simulink model "DCMG_BDCUIO_jan2025_scenario_3"  (R2018b)
settings: Solver=ode1  StartTime=0.0  StopTime=2  FixedStep=1e-6  RelTol=1e-3
undefined symbols (not defined in the file): Cdc, Cpv, dEgdT, EgRef, gcbh, k1, KIvp, KPvp, Rsh_array5pc, sigbuilder_block, sps_rtmsupport, Tref_K, Ts, VT_ref
libraries: powerlib x42, spsPVarrayModel x3
(part 6 of 6)

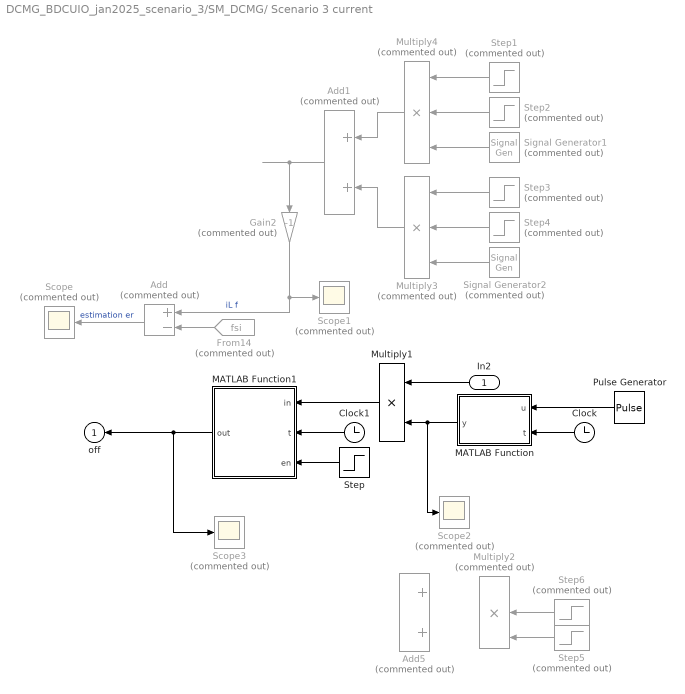
== system DCMG_BDCUIO_jan2025_scenario_3/SM_DCMG/ Scenario 3 current ==
  In2 : Inport
  Add : Sum  Commented=on  Inputs=+-
  Add1 : Sum  Commented=on
  Add5 : Sum  Commented=on
  Clock : Clock
  Clock1 : Clock
  From14 : From  Commented=on  GotoTag=fsi  TagVisibility=global
  Gain2 : Gain  Commented=on  Gain=-1
  MATLAB Function : MATLAB Function  TreatAsAtomicUnit=on
  MATLAB Function1 : MATLAB Function  TreatAsAtomicUnit=on
  Multiply1 : Product
  Multiply2 : Product  Commented=on  Inputs=3
  Multiply3 : Product  Commented=on  Inputs=3
  Multiply4 : Product  Commented=on  Inputs=3
  Pulse Generator : DiscretePulseGenerator  PulseType=Time based  Period=0.01  PulseWidth=40
  Scope{,1..3} (4 alike) : Scope  Commented=on
  Signal Generator1 : SignalGenerator  Commented=on  WaveForm=random  Amplitude=3  Frequency=1100
  Signal Generator2 : SignalGenerator  Commented=on  Amplitude=2  Frequency=25*3.14  Units=rad/sec
  Step : Step  Time=1.1  Before=1  After=0  SampleTime=0
  Step1 : Step  Commented=on  Time=1.1  Before=1  After=0  SampleTime=0
  Step2 : Step  Commented=on  Time=0.7  SampleTime=0
  Step3 : Step  Commented=on  Time=1.7  Before=1  After=0  SampleTime=0
  Step4 : Step  Commented=on  Time=1.2  SampleTime=0
  Step5 : Step  Commented=on  Time=0.5  Before=1  After=0  SampleTime=0
  Step6 : Step  Commented=on  Time=0.25  SampleTime=0
  off : Outport
  wires:
  MATLAB Function/1(y) -> Multiply1/2, Scope2/1
  Clock1/1 -> MATLAB Function1/2(t)
  Step/1 -> MATLAB Function1/3(en)
  MATLAB Function1/1(out) -> off/1, Scope3/1
  Clock/1 -> MATLAB Function/2(t)
  Step6/1 -> Multiply2/2
  Step5/1 -> Multiply2/3
  Pulse Generator/1 -> MATLAB Function/1(u)
  From14/1 -> Add/2
  Add/1 -> Scope/1  "estimation er"
  Signal Generator2/1 -> Multiply3/3
  Step4/1 -> Multiply3/2
  Step3/1 -> Multiply3/1
  Step2/1 -> Multiply4/2
  Step1/1 -> Multiply4/1
  Gain2/1 -> Add/1, Scope1/1  "iL f"
  Add1/1 -> Gain2/1
  Multiply3/1 -> Add1/2
  Multiply4/1 -> Add1/1
  Signal Generator1/1 -> Multiply4/3
  In2/1 -> Multiply1/1
  Multiply1/1 -> MATLAB Function1/1(in)

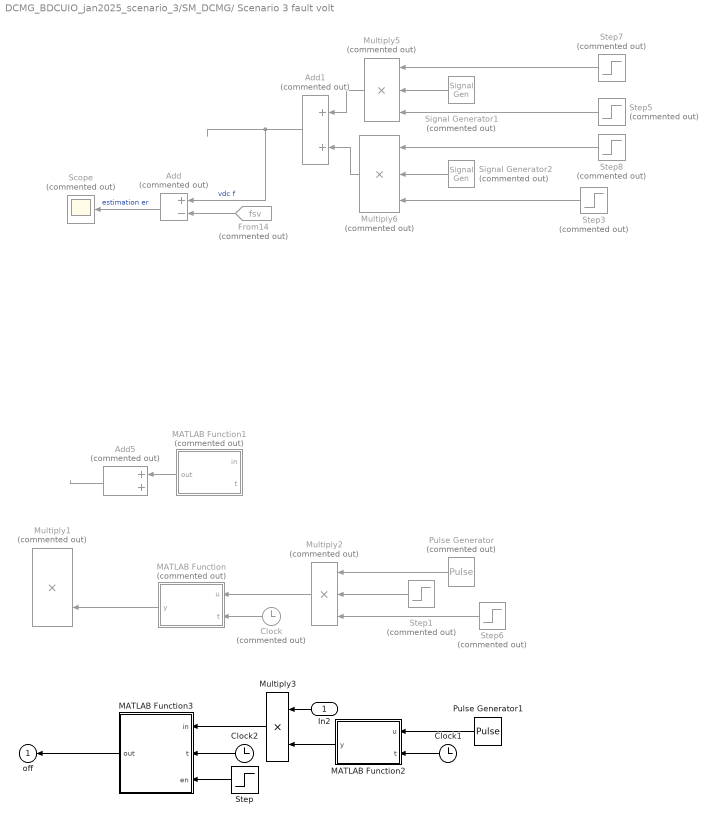
== system DCMG_BDCUIO_jan2025_scenario_3/SM_DCMG/ Scenario 3 fault volt ==
  In2 : Inport
  Add : Sum  Commented=on  Inputs=+-
  Add1 : Sum  Commented=on
  Add5 : Sum  Commented=on
  Clock : Clock  Commented=on
  Clock1 : Clock
  Clock2 : Clock
  From14 : From  Commented=on  GotoTag=fsv  TagVisibility=global
  MATLAB Function : MATLAB Function  Commented=on  TreatAsAtomicUnit=on
  MATLAB Function1 : MATLAB Function  Commented=on  TreatAsAtomicUnit=on
  MATLAB Function2 : MATLAB Function  TreatAsAtomicUnit=on
  MATLAB Function3 : MATLAB Function  TreatAsAtomicUnit=on
  Multiply1 : Product  Commented=on
  Multiply2 : Product  Commented=on  Inputs=3
  Multiply3 : Product
  Multiply5 : Product  Commented=on  Inputs=3
  Multiply6 : Product  Commented=on  Inputs=3
  Pulse Generator : DiscretePulseGenerator  Commented=on  PulseType=Time based  Period=0.1  PulseWidth=30
  Pulse Generator1 : DiscretePulseGenerator  PulseType=Time based  Period=0.01  PulseWidth=40
  Scope : Scope  Commented=on
  Signal Generator1 : SignalGenerator  Commented=on  Amplitude=16  Frequency=45*3.14
  Signal Generator2 : SignalGenerator  Commented=on  WaveForm=random  Amplitude=14  Frequency=5400  Units=rad/sec
  Step : Step  Time=1.7  Before=1  After=0  SampleTime=0
  Step1 : Step  Commented=on  Time=1.7  Before=1  After=0  SampleTime=0
  Step3 : Step  Commented=on  Time=1.2  SampleTime=0
  Step5 : Step  Commented=on  Time=0.2  SampleTime=0
  Step6 : Step  Commented=on  Time=1.2  SampleTime=0
  Step7 : Step  Commented=on  Time=0.6  Before=1  After=0  SampleTime=0
  Step8 : Step  Commented=on  Time=1.7  Before=1  After=0  SampleTime=0
  off : Outport
  wires:
  MATLAB Function2/1(y) -> Multiply3/2
  Step/1 -> MATLAB Function3/3(en)
  Clock1/1 -> MATLAB Function2/2(t)
  Pulse Generator1/1 -> MATLAB Function2/1(u)
  Clock2/1 -> MATLAB Function3/2(t)
  Multiply3/1 -> MATLAB Function3/1(in)
  Step1/1 -> Multiply2/2
  Step3/1 -> Multiply6/3
  MATLAB Function1/1(out) -> Add5/1
  MATLAB Function3/1(out) -> off/1
  MATLAB Function/1(y) -> Multiply1/2
  Clock/1 -> MATLAB Function/2(t)
  Pulse Generator/1 -> Multiply2/1
  Multiply2/1 -> MATLAB Function/1(u)
  Add/1 -> Scope/1  "estimation er"
  From14/1 -> Add/2
  Signal Generator1/1 -> Multiply5/2
  Step7/1 -> Multiply5/1
  Step5/1 -> Multiply5/3
  Add1/1 -> Add/1  "vdc f"
  Step8/1 -> Multiply6/1
  Signal Generator2/1 -> Multiply6/2
  Step6/1 -> Multiply2/3
  Multiply5/1 -> Add1/1
  Multiply6/1 -> Add1/2
  Add5/1 -> ?
  In2/1 -> Multiply3/1

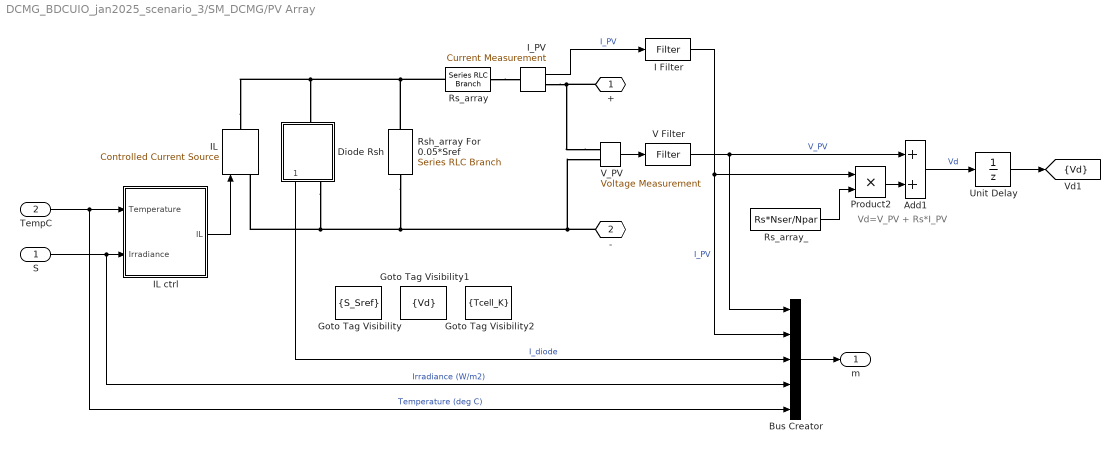
== system DCMG_BDCUIO_jan2025_scenario_3/SM_DCMG/PV Array ==
  note: Vd=V_PV + Rs*I_PV
  S : Inport
  TempC : Inport  Port=2
  Add1 : Sum
  Bus Creator : BusCreator  Inputs=5
  Diode Rsh : Subsystem
      mask Display:
      | plot(-75,-50,100,150, [-15 -15 43 -15 -15 -75],[50 8 50 92 50 50], ...
      |     [43 43],[8 94],[100 43], [50 50])
  Goto Tag Visibility : GotoTagVisibility  GotoTag=S_Sref
  Goto Tag Visibility1 : GotoTagVisibility  GotoTag=Vd
  Goto Tag Visibility2 : GotoTagVisibility  GotoTag=Tcell_K
  I Filter : spsPVarrayModel/Filter  SystemSampleTime=-1  VariantControl=Variant1
  IL : powerlib/Electrical Sources/Controlled Current Source  Initialize=on  Source_Type=AC  Amplitude=0  Phase=0  Frequency=0  Measurements=None
      settings: SourceProductName=Simscape Electrical
  IL ctrl : Subsystem
  I_PV : powerlib/Measurements/Current Measurement  PhasorSimulation=off  OutputType=Complex  PSBequivalent=0
      settings: SourceProductName=Simscape Electrical
  Product2 : Product  Inputs=**  RndMeth=Zero
  Rs_array : powerlib/Elements/Series RLC Branch  LConnTagsString=__new0  RConnTagsString=__new0  BranchType=R  Resistance=Rs*Nser/Npar  Inductance=1e-3  SetiL0=off  InitialCurrent=0  Capacitance=1e-6  Setx0=off  InitialVoltage=0  Measurements=None
      settings: SourceProductName=Simscape Electrical
  Rs_array_ : Constant  Value=Rs*Nser/Npar
  Rsh_array For 0.05*Sref : powerlib/Elements/Series RLC Branch  LConnTagsString=__new0  RConnTagsString=__new0  BranchType=R  Resistance=Rsh_array5pc  Inductance=1e-3  SetiL0=off  InitialCurrent=0  Capacitance=1e-6  Setx0=off  InitialVoltage=0  Measurements=None
      settings: SourceProductName=Simscape Electrical
  Unit Delay : UnitDelay  SampleTime=-1
  V Filter : spsPVarrayModel/Filter  SystemSampleTime=-1  VariantControl=Variant1
  V_PV : powerlib/Measurements/Voltage Measurement  PhasorSimulation=off  OutputType=Complex  PSBequivalent=0
      settings: SourceProductName=Simscape Electrical
  + : PMIOPort  Side=Right
  - : PMIOPort  Port=2  Side=Right
  m : Outport
  tag scope: Vd=scoped
  wires:
  V Filter/1 -> Add1/1, Bus Creator/1  "V_PV"
  I Filter/1 -> Product2/1, Bus Creator/2  "I_PV"
  V_PV/1 -> V Filter/1
  IL ctrl/1(IL) -> IL/1
  Bus Creator/1 -> m/1
  Rs_array_/1 -> Product2/2
  Product2/1 -> Add1/2
  I_PV/1 -> I Filter/1  "I_PV"
  Add1/1 -> Unit Delay/1  "Vd"
  Diode Rsh/1(Idiode) -> Bus Creator/3  "I_diode"
  S/1 -> Bus Creator/4, IL ctrl/2(Irradiance)  "Irradiance (W/m2)"
  TempC/1 -> IL ctrl/1(Temperature), Bus Creator/5  "Temperature (deg C)"
  Unit Delay/1 -> [Vd]
  connections:
  Rs_array/RConn1 -- I_PV/LConn1
  IL/LConn1 -- Diode Rsh/RConn1 -- Rsh_array For 0.05*Sref/RConn1 -- -/RConn1 -- V_PV/LConn2
  IL/RConn1 -- Rsh_array For 0.05*Sref/LConn1 -- Rs_array/LConn1 -- Diode Rsh/LConn1
  V_PV/LConn1 -- I_PV/RConn1 -- +/RConn1

== system DCMG_BDCUIO_jan2025_scenario_3/SM_DCMG/Signal Builder1 ==
  Demux : Demux  Tag=STV Demux  Outputs=1
  FromWs : FromWorkspace  Tag=STV FromWs  VariableName=tuvar  SampleTime=0
      SigBuilderData=|
      | common.afterFinalStr = 'Extrapolate'
      | common.sampleTime = 0
      | dataSet.timeRange = [0 10]
      | dataSet.name = 'Group 1'
      | sbobj.Groups.Name = 'Group 1'
      | sbobj.Groups.Signals.Name = 'Signal 1'
      | sbobj.Groups.Signals.XData = [0 0.96 0.96 2.02 10]
      | sbobj.Groups.Signals.YData = [0.145 0.685 0.68 0.095 0.945]
  Signal 1 : Outport  Tag=STV Outport
  wires:
  Demux/1 -> Signal 1/1
  FromWs/1 -> Demux/1

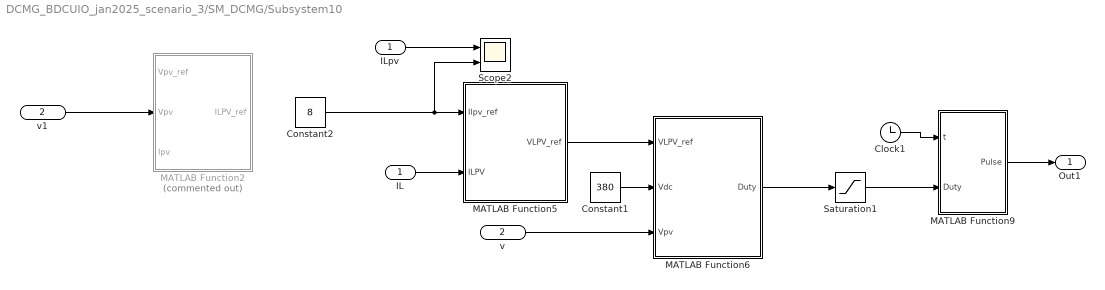
== system DCMG_BDCUIO_jan2025_scenario_3/SM_DCMG/Subsystem10 ==
  ILpv : Inport
  v : Inport  Port=2
  Clock1 : Clock
  Constant1 : Constant  Value=380
  Constant2 : Constant  Value=8
  IL : InportShadow
  MATLAB Function2 : MATLAB Function  Commented=on  TreatAsAtomicUnit=on
  MATLAB Function5 : MATLAB Function  TreatAsAtomicUnit=on
  MATLAB Function6 : MATLAB Function  TreatAsAtomicUnit=on
  MATLAB Function9 : MATLAB Function  TreatAsAtomicUnit=on
  Saturation1 : Saturate  UpperLimit=1  LowerLimit=0
  Scope2 : Scope  NumInputPorts=2
  v1 : InportShadow  Port=2
  Out1 : Outport
  wires:
  Constant1/1 -> MATLAB Function6/2(Vdc)
  v/1 -> MATLAB Function6/3(Vpv)
  ILpv/1 -> Scope2/1
  MATLAB Function6/1(Duty) -> Saturation1/1
  Constant2/1 -> MATLAB Function5/1(Ilpv_ref), Scope2/2
  MATLAB Function5/1(VLPV_ref) -> MATLAB Function6/1(VLPV_ref)
  Clock1/1 -> MATLAB Function9/1(t)
  MATLAB Function9/1(Pulse) -> Out1/1
  Saturation1/1 -> MATLAB Function9/2(Duty)
  v1/1 -> MATLAB Function2/2(Vpv)
  IL/1 -> MATLAB Function5/2(ILPV)

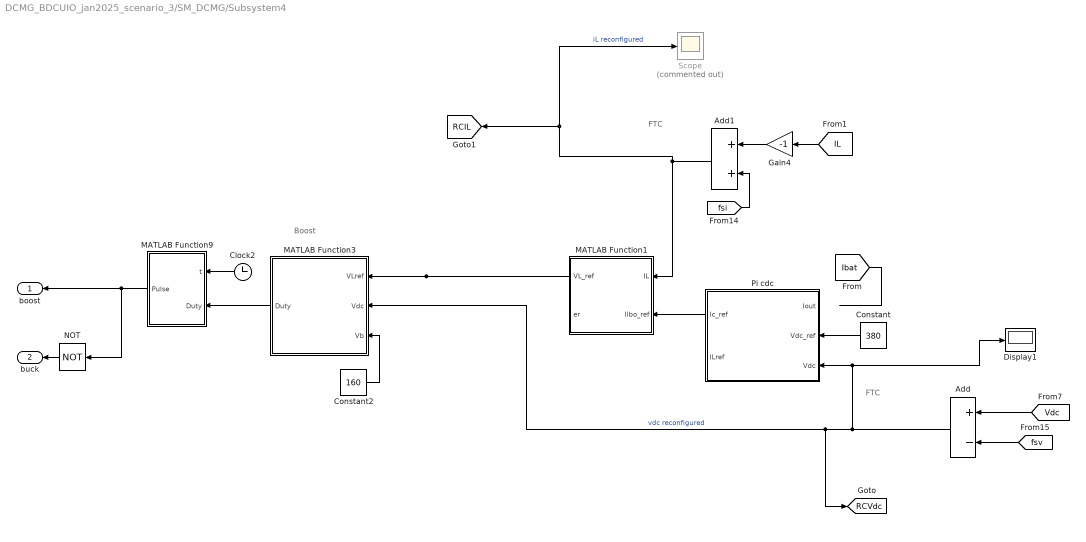
== system DCMG_BDCUIO_jan2025_scenario_3/SM_DCMG/Subsystem4 ==
  note: FTC
  note: Boost
  note: FTC
  Add : Sum  Inputs=+-
  Add1 : Sum
  Clock2 : Clock
  Constant : Constant  Value=380
  Constant2 : Constant  Value=160
  Display1 : Display
  Gain4 : Gain  Gain=-1
  MATLAB Function1 : MATLAB Function  TreatAsAtomicUnit=on
  MATLAB Function3 : MATLAB Function  TreatAsAtomicUnit=on
  MATLAB Function9 : MATLAB Function  TreatAsAtomicUnit=on
  NOT : Logic  Operator=NOT  IconShape=distinctive  AllPortsSameDT=off  OutDataTypeStr=boolean
  Pi cdc : MATLAB Function  TreatAsAtomicUnit=on
  Scope : Scope  Commented=on
  boost : Outport
  buck : Outport  Port=2
  tag scope: RCIL=global, RCVdc=global
  wires:
  MATLAB Function9/1(Pulse) -> NOT/1, boost/1
  MATLAB Function3/1(Duty) -> MATLAB Function9/2(Duty)
  Clock2/1 -> MATLAB Function9/1(t)
  MATLAB Function1/1(VL_ref) -> MATLAB Function3/1(VLref)
  Pi cdc/1(Ic_ref) -> MATLAB Function1/2(Ilbo_ref)
  Constant/1 -> Pi cdc/2(Vdc_ref)
  NOT/1 -> buck/1
  [Vdc] -> Add/1
  [fsv] -> Add/2
  [IL] -> Gain4/1
  [fsi] -> Add1/2
  Add/1 -> Display1/1, Pi cdc/3(Vdc), [RCVdc], MATLAB Function3/2(Vdc)  "vdc reconfigured"
  [Ibat] -> ?
  Constant2/1 -> MATLAB Function3/3(Vb)
  Gain4/1 -> Add1/1
  Add1/1 -> Scope/1, [RCIL], MATLAB Function1/1(IL)  "iL reconfigured"

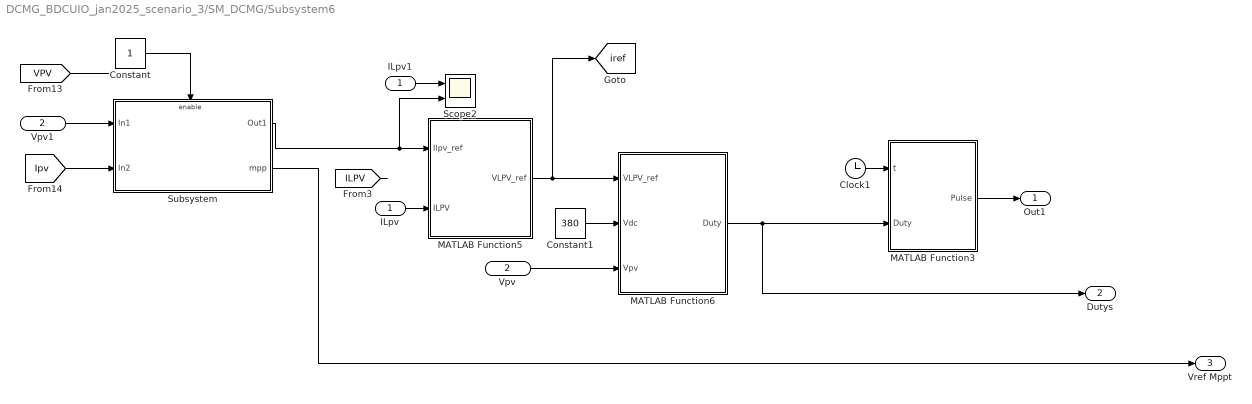
== system DCMG_BDCUIO_jan2025_scenario_3/SM_DCMG/Subsystem6 ==
  ILpv : Inport
  Vpv : Inport  Port=2
  Clock1 : Clock
  Constant : Constant
  Constant1 : Constant  Value=380
  ILpv1 : InportShadow
  MATLAB Function3 : MATLAB Function  TreatAsAtomicUnit=on
  MATLAB Function5 : MATLAB Function  TreatAsAtomicUnit=on
  MATLAB Function6 : MATLAB Function  TreatAsAtomicUnit=on
  Scope2 : Scope  NumInputPorts=2
  Subsystem : Subsystem
  Vpv1 : InportShadow  Port=2
  Out1 : Outport
  Dutys : Outport  Port=2
  Vref Mppt : Outport  Port=3
  tag scope: iref=global
  wires:
  MATLAB Function3/1(Pulse) -> Out1/1
  Clock1/1 -> MATLAB Function3/1(t)
  [ILPV] -> ?
  MATLAB Function5/1(VLPV_ref) -> [iref], MATLAB Function6/1(VLPV_ref)
  [VPV] -> ?
  [Ipv] -> Subsystem/2(In2)
  Constant/1 -> Subsystem/Enable
  Subsystem/1(Out1) -> Scope2/2, MATLAB Function5/1(Ilpv_ref)
  MATLAB Function6/1(Duty) -> Dutys/1, MATLAB Function3/2(Duty)
  Subsystem/2(mpp) -> Vref Mppt/1
  ILpv/1 -> MATLAB Function5/2(ILPV)
  ILpv1/1 -> Scope2/1
  Vpv/1 -> MATLAB Function6/3(Vpv)
  Vpv1/1 -> Subsystem/1(In1)
  Constant1/1 -> MATLAB Function6/2(Vdc)

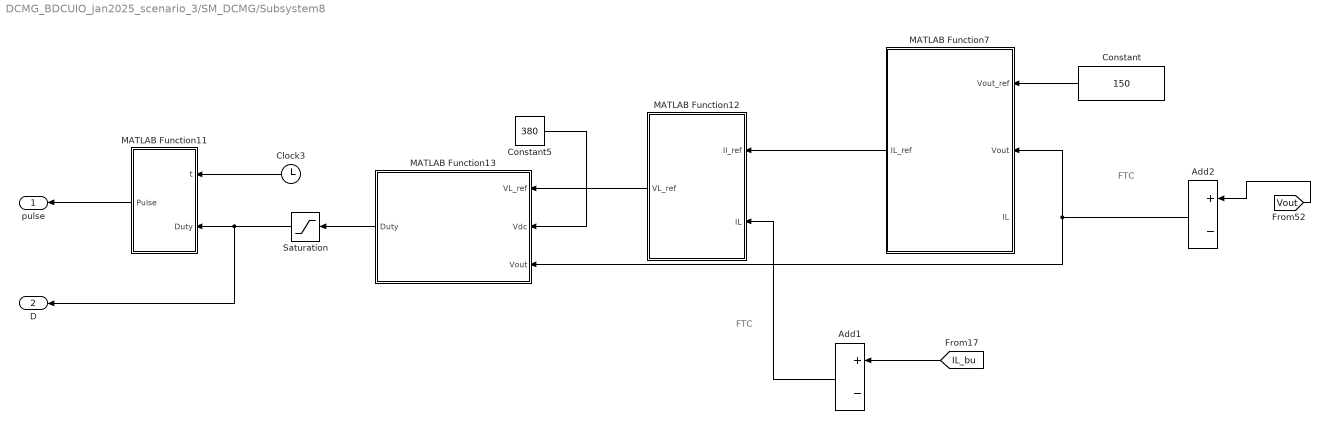
== system DCMG_BDCUIO_jan2025_scenario_3/SM_DCMG/Subsystem8 ==
  note: FTC
  note: FTC
  Add1 : Sum  Inputs=+-
  Add2 : Sum  Inputs=+-
  Clock3 : Clock
  Constant : Constant  Value=150
  Constant5 : Constant  Value=380
  MATLAB Function11 : MATLAB Function  TreatAsAtomicUnit=on
  MATLAB Function12 : MATLAB Function  TreatAsAtomicUnit=on
  MATLAB Function13 : MATLAB Function  TreatAsAtomicUnit=on
  MATLAB Function7 : MATLAB Function  TreatAsAtomicUnit=on
  Saturation : Saturate  UpperLimit=1  LowerLimit=0
  pulse : Outport
  D : Outport  Port=2
  wires:
  MATLAB Function11/1(Pulse) -> pulse/1
  Clock3/1 -> MATLAB Function11/1(t)
  MATLAB Function13/1(Duty) -> Saturation/1
  MATLAB Function7/1(IL_ref) -> MATLAB Function12/1(Il_ref)
  Constant/1 -> MATLAB Function7/1(Vout_ref)
  MATLAB Function12/1(VL_ref) -> MATLAB Function13/1(VL_ref)
  Add2/1 -> MATLAB Function7/2(Vout), MATLAB Function13/3(Vout)
  [IL_bu] -> Add1/1
  Constant5/1 -> MATLAB Function13/2(Vdc)
  Add1/1 -> MATLAB Function12/2(IL)
  Saturation/1 -> MATLAB Function11/2(Duty), D/1
  [Vout] -> Add2/1

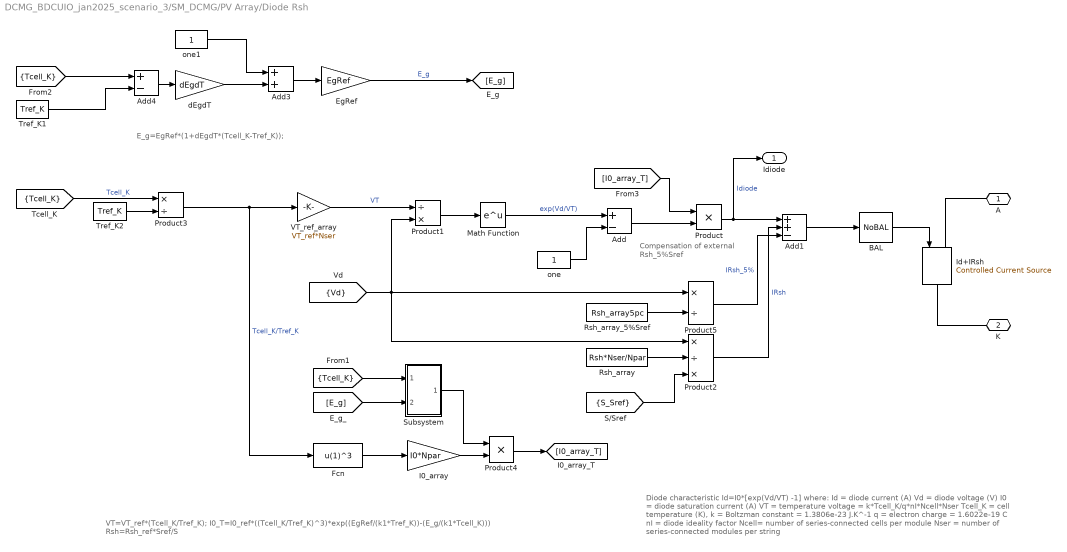
== system DCMG_BDCUIO_jan2025_scenario_3/SM_DCMG/PV Array/Diode Rsh ==
  note: Compensation of
      | external Rsh_5%Sref
  note: Diode characteristic
      |    Id=I0*[exp(Vd/VT) -1]
      |
      | where:
      |      Id = diode current (A)
      |      Vd = diode voltage (V)
      |      I0 = diode saturation current (A)
      |      VT = temperature voltage = k*Tcell_K/q*nI*Ncell*Nser
      | Tcell_K = cell temperature (K),
      |       k = Boltzman constant = 1.3806e-23 J.K^-1
      |       q = electron charge = 1.6022e-19 C
      |      nI = diode ideality factor
      |    Ncell= number of series-connected cells per module
      |    Nser = number of series-connected modules per string
  note: VT=VT_ref*(Tcell_K/Tref_K);
      | I0_T=I0_ref*((Tcell_K/Tref_K)^3)*exp((EgRef/(k1*Tref_K))-(E_g/(k1*Tcell_K)))
      | Rsh=Rsh_ref*Sref/S
  note: E_g=EgRef*(1+dEgdT*(Tcell_K-Tref_K));
  Add : Sum  Inputs=+-
  Add1 : Sum  Inputs=++-
  Add3 : Sum
  Add4 : Sum  Inputs=+-
  BAL : spsPVarrayModel/NoBAL  SystemSampleTime=-1  VariantControl=NoBAL
  EgRef : Gain  Gain=EgRef
  Fcn : Fcn  Expr=u(1)^3
  I0_array : Gain  Gain=I0*Npar
  Id+IRsh : powerlib/Electrical Sources/Controlled Current Source  Initialize=on  Source_Type=AC  Amplitude=0  Phase=0  Frequency=0  Measurements=None
      settings: SourceProductName=Simscape Electrical
  Math Function : Math  SaturateOnIntegerOverflow=on
  Product : Product  RndMeth=Zero
  Product1 : Product  Inputs=/*  RndMeth=Zero
  Product2 : Product  Inputs=*/*  RndMeth=Zero
  Product3 : Product  Inputs=*/  RndMeth=Zero
  Product4 : Product  Inputs=**  RndMeth=Zero
  Product5 : Product  Inputs=*/  RndMeth=Zero
  Rsh_array : Constant  Value=Rsh*Nser/Npar
  Rsh_array_5%Sref : Constant  Value=Rsh_array5pc
  Subsystem : Subsystem
  Tref_K1 : Constant  Value=Tref_K
  Tref_K2 : Constant  Value=Tref_K
  VT_ref_array : Gain  Gain=VT_ref*Nser
  dEgdT : Gain  Gain=dEgdT
  one : Constant
  one1 : Constant
  A : PMIOPort  Side=Left
  K : PMIOPort  Port=2  Side=Right
  Idiode : Outport
  wires:
  BAL/1 -> Id+IRsh/1
  Add1/1 -> BAL/1
  Product5/1 -> Add1/3  "IRsh_5%"
  Rsh_array_5%Sref/1 -> Product5/2
  Math Function/1 -> Add/1  "exp(Vd/VT)"
  Product2/1 -> Add1/2  "IRsh"
  Product/1 -> Add1/1, Idiode/1  "Idiode"
  Product1/1 -> Math Function/1
  one/1 -> Add/2
  Rsh_array/1 -> Product2/2
  [Tcell_K] -> Product3/1  "Tcell_K"
  Product3/1 -> VT_ref_array/1, Fcn/1  "Tcell_K/Tref_K"
  one1/1 -> Add3/1
  Add4/1 -> dEgdT/1
  dEgdT/1 -> Add3/2
  Add3/1 -> EgRef/1
  EgRef/1 -> [E_g]  "E_g"
  I0_array/1 -> Product4/2
  Fcn/1 -> I0_array/1
  [Tcell_K] -> Add4/1
  Tref_K1/1 -> Add4/2
  Subsystem/1(exp) -> Product4/1
  [Tcell_K] -> Subsystem/1(Tcell_K)
  [E_g] -> Subsystem/2(E_g)
  Tref_K2/1 -> Product3/2
  Product4/1 -> [I0_array_T]
  Add/1 -> Product/2
  VT_ref_array/1 -> Product1/1  "VT"
  [I0_array_T] -> Product/1
  [S_Sref] -> Product2/3
  [Vd] -> Product5/1, Product2/1, Product1/2
  connections:
  Id+IRsh/RConn1 -- K/RConn1
  A/RConn1 -- Id+IRsh/LConn1

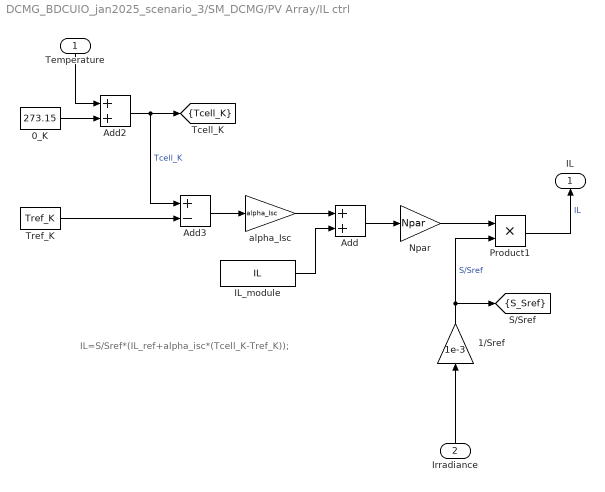
== system DCMG_BDCUIO_jan2025_scenario_3/SM_DCMG/PV Array/IL ctrl ==
  note: IL=S/Sref*(IL_ref+alpha_isc*(Tcell_K-Tref_K));
  Temperature : Inport
  Irradiance : Inport  Port=2
  0_K : Constant  Value=273.15
  1/Sref : Gain  Gain=1e-3
  Add : Sum
  Add2 : Sum
  Add3 : Sum  Inputs=+-
  IL_module : Constant  Value=IL
  Npar : Gain  Gain=Npar
  Product1 : Product  Inputs=**  RndMeth=Zero
  Tref_K : Constant  Value=Tref_K
  alpha_Isc : Gain  Gain=alpha_Isc
  IL : Outport
  tag scope: S_Sref=scoped, Tcell_K=scoped
  wires:
  Temperature/1 -> Add2/1
  Irradiance/1 -> 1/Sref/1
  alpha_Isc/1 -> Add/1
  Add3/1 -> alpha_Isc/1
  Tref_K/1 -> Add3/2
  Product1/1 -> IL/1  "IL"
  IL_module/1 -> Add/2
  0_K/1 -> Add2/2
  Add/1 -> Npar/1
  Add2/1 -> Add3/1, [Tcell_K]  "Tcell_K"
  Npar/1 -> Product1/1
  1/Sref/1 -> Product1/2, [S_Sref]  "S/Sref"

== system DCMG_BDCUIO_jan2025_scenario_3/SM_DCMG/Subsystem6/Subsystem ==
  In1 : Inport
  In2 : Inport  Port=2
  Enable : EnablePort
  MATLAB Function2 : MATLAB Function  TreatAsAtomicUnit=on
  MATLAB Function7 : MATLAB Function  TreatAsAtomicUnit=on
  Scope3 : Scope  NumInputPorts=2
  Out1 : Outport
  mpp : Outport  Port=2
  wires:
  MATLAB Function2/1(ILPV_ref) -> Out1/1
  MATLAB Function7/1(Vref) -> Scope3/1, mpp/1, MATLAB Function2/1(Vpv_ref)
  In1/1 -> Scope3/2, MATLAB Function2/2(Vpv), MATLAB Function7/1(Vpv)
  In2/1 -> MATLAB Function2/3(Ipv), MATLAB Function7/2(Ipv)

== system DCMG_BDCUIO_jan2025_scenario_3/SM_DCMG/PV Array/Diode Rsh/Subsystem ==
  note: exp((EgRef/(k1*Tref_K))-(E_g/(k1*Tcell_K)))
  Tcell_K : Inport
  E_g : Inport  Port=2
  Add : Sum  Inputs=+-
  EgRef : Constant  Value=EgRef/(k1*Tref_K)
  Math Function : Math  SaturateOnIntegerOverflow=on
  Product : Product  Inputs=*/
  k1 : Gain  Gain=k1
  exp : Outport
  wires:
  EgRef/1 -> Add/1
  E_g/1 -> Product/1
  Tcell_K/1 -> k1/1
  k1/1 -> Product/2
  Product/1 -> Add/2
  Add/1 -> Math Function/1
  Math Function/1 -> exp/1

== matlab function DCMG_BDCUIO_jan2025_scenario_3/SM_DCMG/Subsystem6/Subsystem/MATLAB Function2 ==
  data: ILPV_ref output; Vpv_ref input; Vpv input; Ipv input
function ILPV_ref = PI( Vpv_ref,Vpv,Ipv )
%#codegen
Ts=1e-6;
KPvp=0.95125;
KIvp=91;


er=Vpv_ref-Vpv;
% ki=wn_cpv^2*Cpv;
% kp=2*ksi_cpv*wn_cpv*Cpv;
persistent Icpv_past 

if isempty(Icpv_past)
    Icpv_past=0;
end
Icpv_past=Icpv_past+er*Ts;

err_integrated=Icpv_past;

Icpv_ref=KIvp*KPvp*err_integrated+KPvp*er;


ILPV_ref=Ipv-Icpv_ref;

== matlab function DCMG_BDCUIO_jan2025_scenario_3/SM_DCMG/Subsystem6/MATLAB Function5 ==
  settings: updateMethod=DISCRETE
  data: Ilpv_ref input; VLPV_ref output; ILPV input
function VLPV_ref = fcn(Ilpv_ref,ILPV )
%#codegen

Ts=1e-6;
KPpv=9.17758;
KIpv=61;

er=Ilpv_ref-ILPV;

% ki=Lpv*Wnlpv^2;
% kp=2*Lpv*Ksi_lpv*Wnlpv-R_pv;

persistent er_past 
if isempty(er_past)
    er_past=0;
end
er_past=er_past+er*Ts;

err_integrated=er_past;



VLPV_ref = KIpv*KPpv*err_integrated+KPpv*er;

== matlab function DCMG_BDCUIO_jan2025_scenario_3/SM_DCMG/Subsystem10/MATLAB Function5 ==
  settings: updateMethod=DISCRETE
  data: Ilpv_ref input; VLPV_ref output; ILPV input
function VLPV_ref = fcn(Ilpv_ref,ILPV )
%#codegen
Ts=1e-6;
KPpv=9.17758;
KIpv=61;
er=Ilpv_ref-ILPV;

% ki=Lpv*Wnlpv^2;
% kp=2*Lpv*Ksi_lpv*Wnlpv-R_pv;

persistent er_past 
if isempty(er_past)
    er_past=0;
end
er_past=er_past+er*Ts;

err_integrated=er_past;



VLPV_ref = 29*KIpv*KPpv*err_integrated+4*KPpv*er;

== matlab function DCMG_BDCUIO_jan2025_scenario_3/SM_DCMG/Subsystem10/MATLAB Function6 ==
  data: VLPV_ref input; Vdc input; Duty output; Vpv input
function Duty = PI(VLPV_ref,Vdc,Vpv)
%#codegen
% Vdc=380;
 V_ref=Vpv-VLPV_ref;
 D=1-(V_ref/Vdc);
 
 if D > 0.9
 D_limite=0.9;
 elseif D < 0
 D_limite=0;
 else
 D_limite=D;
 end
 Duty=D_limite;
end

== matlab function DCMG_BDCUIO_jan2025_scenario_3/SM_DCMG/ Scenario 3 current/MATLAB Function ==
  data: u input; y output; t input
function y = fcn(u,t)

if t>1.2 && t<1.7
    y=u;
else
    y=1;
end

== matlab function DCMG_BDCUIO_jan2025_scenario_3/SM_DCMG/ Scenario 3 current/MATLAB Function1 ==
  settings: updateMethod=DISCRETE
  data: in input; out output; t input; en input
function out = fnc(in, t,en)

tf=0.7;
persistent lIn; 

if isempty(lIn)
   lIn = in; 
end
if en==1
    if t < tf
    lIn = in;
    out = in; % Output current input
    else
    out = lIn; % Output last recorded input
    end
else
    lIn = in;
    out = in; % Output current input
end
end

== matlab function DCMG_BDCUIO_jan2025_scenario_3/SM_DCMG/Subsystem6/MATLAB Function6 ==
  data: VLPV_ref input; Vdc input; Duty output; Vpv input
function Duty = PI(VLPV_ref,Vdc,Vpv)
%#codegen
% Vdc=380;
 V_ref=Vpv-VLPV_ref;
 D=1-(V_ref/Vdc);
 
 if D > 0.9
 D_limite=0.9;
 elseif D < 0
 D_limite=0;
 else
 D_limite=D;
 end
 Duty=D_limite;
end

== matlab function DCMG_BDCUIO_jan2025_scenario_3/SM_DCMG/Subsystem6/Subsystem/MATLAB Function7 ==
  settings: updateMethod=DISCRETE  sampleTime=100*1e-6
  data: Vpv input; Vref output; Ipv input
function Vref = PnO(Vpv,Ipv)
DeltaVpv_ref=2;
% DeltaVpv_ref=0.5;
persistent Vold ;
if isempty(Vold)
Vold=0;
end
persistent Pold ;
if isempty(Pold)
Pold=0;
end
P= Vpv*Ipv;
dV= Vpv - Vold;
dP= P - Pold;

if dP>0
    if dV>0
         Vref=Vold+DeltaVpv_ref;
    else
         Vref=Vold-DeltaVpv_ref;
    end
elseif dP<0
     if dV>0
         Vref=Vold-DeltaVpv_ref;
    else
         Vref=Vold+DeltaVpv_ref;
     end
else
    Vref=Vold;
end



Vold=Vpv;
Pold=P;

== matlab function DCMG_BDCUIO_jan2025_scenario_3/SM_DCMG/Subsystem8/MATLAB Function11 ==
  data: t input; Pulse output; Duty input
function Pulse = PWM(t,Duty)
%#codegen
fs=40e3;
Te=1/fs;
 tt=mod(t,Te);
 if(tt<Duty*Te)
 S=1;
 else
 S=0;
 end
 Pulse= S;

== matlab function DCMG_BDCUIO_jan2025_scenario_3/SM_DCMG/Subsystem8/MATLAB Function12 ==
  settings: updateMethod=DISCRETE
  data: Il_ref input; VL_ref output; IL input
function VL_ref = fcn(Il_ref,IL )
%#codegen

Ts=1e-6;

er=Il_ref-IL;Wn_lbu=300;
Ksi_lbu=0.9;
 R_bu=0.0001;L_bu=7e-3;
ki=L_bu*Wn_lbu^2;
kp=2*L_bu*Ksi_lbu*Wn_lbu-R_bu;

persistent er_past 
if isempty(er_past)
    er_past=0;
end
er_past=er_past+er*Ts;

err_integrated=er_past;

VL_ref = ki*err_integrated+kp*er;

% VL_ref = kP*kI*err_integrated+kP*er;

== matlab function DCMG_BDCUIO_jan2025_scenario_3/SM_DCMG/Subsystem8/MATLAB Function13 ==
  data: VL_ref input; Vdc input; Duty output; Vout input
function Duty = duty(VL_ref,Vdc,Vout)
%#codegen
%  Vs_ref=Vout+VL_ref;
%  V_ref=Vs_ref-VL_ref;
Vref=VL_ref+Vout;
 D=(Vref/Vdc);
 if D > 0.9
 D_limite=0.9;
 elseif D < 0
 D_limite=0;
 else
 D_limite=D;
 end
 Duty=D_limite;
end

== matlab function DCMG_BDCUIO_jan2025_scenario_3/SM_DCMG/Subsystem8/MATLAB Function7 ==
  settings: updateMethod=DISCRETE
  data: IL_ref output; Vout_ref input; Vout input; IL input
function IL_ref = PI( Vout_ref,Vout,IL )
%#codegen
Ts=1e-6;
er=Vout_ref-Vout;
ksi_bu=0.707;
wn_bu=150;
Cout=35.5e-04;
ki=wn_bu^2*Cout;
kp=2*ksi_bu*wn_bu*Cout;
persistent Ic_past 

if isempty(Ic_past)
    Ic_past=0;
end
Ic_past=Ic_past+er*Ts;

err_integrated=Ic_past;

Ic_ref=ki*err_integrated+kp*er;

% Ic_ref=kPv*kIv*err_integrated+kPv*er;

% IL_ref=Ic_ref;
IL_ref=IL+Ic_ref;

== matlab function DCMG_BDCUIO_jan2025_scenario_3/SM_DCMG/ Scenario 3 fault volt/MATLAB Function ==
  data: u input; y output; t input
function y = fcn(u,t)

if t<0.5 && t>0.25
    y=u;
else
    y=1;
end

== matlab function DCMG_BDCUIO_jan2025_scenario_3/SM_DCMG/Subsystem10/MATLAB Function2 ==
  data: Ts parameter; ILPV_ref output; Vpv_ref input; Vpv input; Ipv input; KIvp parameter; Cpv parameter; KPvp parameter
function ILPV_ref = PI( Ts,Vpv_ref,Vpv,Ipv,KIvp,Cpv,KPvp)
%#codegen

er=Vpv_ref-Vpv;
% ki=wn_cpv^2*Cpv;
% kp=2*ksi_cpv*wn_cpv*Cpv;
persistent Icpv_past 

if isempty(Icpv_past)
    Icpv_past=0;
end
Icpv_past=Icpv_past+er*Ts;

err_integrated=Icpv_past;

Icpv_ref=KIvp*KPvp*err_integrated+KPvp*er;


ILPV_ref=Ipv-Icpv_ref;

== matlab function DCMG_BDCUIO_jan2025_scenario_3/SM_DCMG/Subsystem4/MATLAB Function1 ==
  settings: updateMethod=DISCRETE
  data: VL_ref output; IL input; Ilbo_ref input; er output
function [VL_ref,er]= fcn(IL,Ilbo_ref )
%#codegen
Ts=1e-6;
R_b=0.016;
L_b=0.012;
Wn_B=390;
Ksi_B=0.8;
    er=Ilbo_ref-IL;

% 
ki=L_b*Wn_B^2;
kp=2*L_b*Ksi_B*Wn_B-R_b;

% ki=0.002;
% kp=0.002;
persistent er_past 
if isempty(er_past)
    er_past=0;
end
er_past=er_past+er*Ts;

err_integrated=er_past;



VL_ref =ki*err_integrated+kp*er;

== matlab function DCMG_BDCUIO_jan2025_scenario_3/SM_DCMG/Subsystem4/MATLAB Function3 ==
  data: VLref input; Vdc input; Duty output; Vb input
function Duty= fnc(VLref,Vdc,Vb)
%#codegen


% if Iref >= 0
%    D=0;
% else
    Vref=Vb+VLref;
   D=1-(Vref/Vdc);
% end
 if D > 0.9
 D_limite=0.9;
 elseif D < 0
 D_limite=0;
 else
 D_limite=D;
 end
 Duty=D_limite;
end

== matlab function DCMG_BDCUIO_jan2025_scenario_3/SM_DCMG/Subsystem10/MATLAB Function9 ==
  data: t input; Pulse output; Duty input
function Pulse = PWM(t,Duty)
%#codegen
fs=25e3;
 Te=1/fs;
 tt=mod(t,Te);
 if(tt<Duty*Te)
 S=1;
 else
 S=0;
 end
 Pulse= S;

== matlab function DCMG_BDCUIO_jan2025_scenario_3/SM_DCMG/ Scenario 3 fault volt/MATLAB Function1 ==
  settings: updateMethod=DISCRETE
  data: in input; out output; t input
function out = fnc(in, t)

tf=0.6;
persistent lIn; 

if isempty(lIn)
   lIn = in; 
end

    
if t < tf
    lIn = in;
    out = in; % Output current input
else
    out = lIn; % Output last recorded input
end
end

== matlab function DCMG_BDCUIO_jan2025_scenario_3/SM_DCMG/Subsystem4/MATLAB Function9 ==
  data: t input; Pulse output; Duty input
function Pulse = PWM(t,Duty)
%#codegen
fs=25e3;
 Te=1/fs;
 tt=mod(t,Te);
 if(tt<Duty*Te)
 S=1;
 else
 S=0;
 end
 Pulse= S;

== matlab function DCMG_BDCUIO_jan2025_scenario_3/SM_DCMG/Subsystem4/Pi cdc ==
  settings: updateMethod=DISCRETE
  data: Iout input; Vdc_ref input; Vdc input; Ic_ref output; ILref output
function [Ic_ref ,ILref]= PI(Iout, Vdc_ref,Vdc )
%#

Ts=1e-6;
ksi=0.7;
Wn=220;
Cdc=900e-06;
er=Vdc-Vdc_ref;


ki=Wn^2*Cdc;
kp=2*ksi*Wn*Cdc;
persistent Ic_past 

if isempty(Ic_past)
    Ic_past=0;
end
Ic_past=Ic_past+er*Ts;

err_integrated=Ic_past;

Ic_ref= ki*err_integrated+kp*er;

ILref=Ic_ref+Iout;

== matlab function DCMG_BDCUIO_jan2025_scenario_3/SM_DCMG/ Scenario 3 fault volt/MATLAB Function2 ==
  data: u input; y output; t input
function y = fcn(u,t)

if t>0.2 && t<0.6
    y=u;
else
    y=1;
end

== matlab function DCMG_BDCUIO_jan2025_scenario_3/SM_DCMG/ Scenario 3 fault volt/MATLAB Function3 ==
  settings: updateMethod=DISCRETE
  data: in input; out output; t input; en input
function out = fnc(in, t,en)

tf=1.2;
persistent lIn; 

if isempty(lIn)
   lIn = in; 
end
if en==1
    if t < tf
    lIn = in;
    out = in; % Output current input
    else
    out = lIn; % Output last recorded input
    end
else
    lIn = in;
    out = in; % Output current input
end
end

== matlab function DCMG_BDCUIO_jan2025_scenario_3/SM_DCMG/ Ui-PIO3 ==
  settings: updateMethod=DISCRETE
  data: xhat1 output; Vin input; iload input; X input; xhat2 output; xhat3 output; xhat4 output; s input
function [xhat1,xhat2,xhat3,xhat4]=  Ui_PIO(Vin,iload,X, s)


Ts=1e-6;
Cbar=eye(2);
C=[Cbar eye(2)];
Kss =[5.45074961823853954001606325619 -0.000507925775440352337414262606785;-0.0182932753131756706266308754039 3.76757255202677665550936580985;6.76571201159828383708827459486 0.00268839100561887043086550797;0.0170561761430559136187845581389 8.45313029348350397640388109721];
T1 =[1 0 0 0;0 1 0 0;-1 0 0 0;0 -1 0 0];
T2 =[-1.18387322150443e-16 0;0 -1.18387322150443e-16;1 0;0 1];

G =[83.3333333333332859638176159933 0;0 -1111.11111111111063110001850873;-83.3333333333333001746723311953 0;0 1111.11111111111063110001850873];



Cdc=900e-06;
%% % Bi DC-DC converter
R_b=0.016;
L_b=0.012;

persistent z1
if isempty(z1)
    z1=00;
end
persistent z2
if isempty(z2)
    z2=380;
end
persistent z3
if isempty(z3)
    z3=0;
end
persistent z4
if isempty(z4)
    z4=-380;
end
Z=[z1;z2;z3;z4];
u=[Vin;iload];
y=C*X;
Abar=[-R_b/L_b -(1-s)/(L_b) ;
    (1-s)/Cdc  0];

A=[Abar zeros(2,2);
    zeros(2,2) -eye(2)];
Ns=T1*A-Kss*C;
Ls=Kss+Ns*T2;

Zdot=Ns*Z+G*u+Ls*y;
Z=Z+ Zdot*Ts;
xhat=Z+T2*y;

z1=Z(1,1);
z2=Z(2,:);
z3=Z(3,:);
z4=Z(4,:);
xhat1=xhat(1,1);
xhat2=xhat(2,1);
xhat3=xhat(3,1);
xhat4=xhat(4,1);
end

== matlab function DCMG_BDCUIO_jan2025_scenario_3/SM_DCMG/Subsystem6/MATLAB Function3 ==
  data: t input; Pulse output; Duty input
function Pulse = PWM(t,Duty)
%#codegen
fs=55e3;
Te=1/fs;
 tt=mod(t,Te);
 if(tt<Duty*Te)
 S=1;
 else
 S=0;
 end
 Pulse= S;
